simulink model "MCU_Input"  (R2022b)
settings: Solver=FixedStepDiscrete  StartTime=0.0  StopTime=10.0  FixedStep=1e-4  RelTol=1e-3
values from neighbouring files (symbols this model uses):
  C_ADC_Acc1Offset_i32 = 0.0    [MCU_Input_Sldd.sldd]    (also in MCU_Input_Sldd_objects.m = myPackage.Parameter)
  C_ADC_BrakeOffset_i32 = 0.0    [MCU_Input_Sldd.sldd]    (also in MCU_Input_Sldd_objects.m = myPackage.Parameter)
  C_ADC_HSTempGain_f32 = 0.0    [MCU_Input_Sldd.sldd]    (also in MCU_Input_Sldd_objects.m = myPackage.Parameter)
  C_ADC_HSTempOffset_i32 = 0.0    [MCU_Input_Sldd.sldd]    (also in MCU_Input_Sldd_objects.m = myPackage.Parameter)
  C_ADC_IdcOffset_i32 = 0.0    [MCU_Input_Sldd.sldd]    (also in MCU_Input_Sldd_objects.m = myPackage.Parameter)
  C_ADC_IGBTTable_i16 = 0.0    [MCU_Input_Sldd.sldd]    (also in MCU_Input_Sldd_objects.m = myPackage.Parameter)
  C_ADC_IGBTTempGain_f32 = 0.0    [MCU_Input_Sldd.sldd]    (also in MCU_Input_Sldd_objects.m = myPackage.Parameter)
  C_ADC_IGBTTempOffset_i32 = 0.0    [MCU_Input_Sldd.sldd]    (also in MCU_Input_Sldd_objects.m = myPackage.Parameter)
  C_ADC_MotorTemp1Gain_f32 = 0.0    [MCU_Input_Sldd.sldd]    (also in MCU_Input_Sldd_objects.m = myPackage.Parameter)
  C_ADC_MotorTemp1Offset_i32 = 0.0    [MCU_Input_Sldd.sldd]    (also in MCU_Input_Sldd_objects.m = myPackage.Parameter)
  C_ADC_MotorTempTable_i16 = 0.0    [MCU_Input_Sldd.sldd]    (also in MCU_Input_Sldd_objects.m = myPackage.Parameter)
  C_ADC_P12VOffset_i32 = 0.0    [MCU_Input_Sldd.sldd]    (also in MCU_Input_Sldd_objects.m = myPackage.Parameter)
  C_ADC_P15VOffset_i32 = 0.0    [MCU_Input_Sldd.sldd]    (also in MCU_Input_Sldd_objects.m = myPackage.Parameter)
  C_ADC_P5VOffset_i32 = 0.0    [MCU_Input_Sldd.sldd]    (also in MCU_Input_Sldd_objects.m = myPackage.Parameter)
  C_DCCurrent_DrvCoeff_f32 = 0.0    [MCU_Input_Sldd.sldd]    (also in MCU_Input_Sldd_objects.m = myPackage.Parameter)
  C_DCCurrent_GenCoeff_f32 = 0.0    [MCU_Input_Sldd.sldd]    (also in MCU_Input_Sldd_objects.m = myPackage.Parameter)
  C_Encoder_CurrentAdder_f32 = 0.0    [MCU_Input_Sldd.sldd]    (also in MCU_Input_Sldd_objects.m = myPackage.Parameter)
  C_Encoder_WaitTime_f32 = 0.0    [MCU_Input_Sldd.sldd]    (also in MCU_Input_Sldd_objects.m = myPackage.Parameter)
  C_Input_EncErr_u8 = 0.0    [MCU_Input_Sldd.sldd]    (also in MCU_Input_Sldd_objects.m = myPackage.Parameter)
  C_Rotate_RotateBits_u8 = 0.0    [MCU_Input_Sldd.sldd]    (also in MCU_Input_Sldd_objects.m = myPackage.Parameter)
  C_Rotate_SetAngle_u16 = 0.0    [MCU_Input_Sldd.sldd]    (also in MCU_Input_Sldd_objects.m = myPackage.Parameter)
  C_Rotate_SetAngleFlg_u8 = 0.0    [MCU_Input_Sldd.sldd]    (also in MCU_Input_Sldd_objects.m = myPackage.Parameter)
  C_SelfCheck_AvgCntSet_u16 = 0.0    [MCU_Input_Sldd.sldd]    (also in MCU_Input_Sldd_objects.m = myPackage.Parameter)
  C_SelfCheck_DelayTimeSet_u16 = 0.0    [MCU_Input_Sldd.sldd]    (also in MCU_Input_Sldd_objects.m = myPackage.Parameter)
  C_SelfCheck_IaoffsetDownLimt_u16 = 0.0    [MCU_Input_Sldd.sldd]    (also in MCU_Input_Sldd_objects.m = myPackage.Parameter)
  C_SelfCheck_IaoffsetUpLimt_u16 = 0.0    [MCU_Input_Sldd.sldd]    (also in MCU_Input_Sldd_objects.m = myPackage.Parameter)
  C_SelfCheck_IboffsetDownLimt_u16 = 0.0    [MCU_Input_Sldd.sldd]    (also in MCU_Input_Sldd_objects.m = myPackage.Parameter)
  C_SelfCheck_IboffsetUpLimt_u16 = 0.0    [MCU_Input_Sldd.sldd]    (also in MCU_Input_Sldd_objects.m = myPackage.Parameter)
  C_SelfCheck_IcoffsetDownLimt_u16 = 0.0    [MCU_Input_Sldd.sldd]    (also in MCU_Input_Sldd_objects.m = myPackage.Parameter)
  C_SelfCheck_IcoffsetUpLimt_u16 = 0.0    [MCU_Input_Sldd.sldd]    (also in MCU_Input_Sldd_objects.m = myPackage.Parameter)
  C_SelfCheck_OffsetUnCal_u8 = 0.0    [MCU_Input_Sldd.sldd]    (also in MCU_Input_Sldd_objects.m = myPackage.Parameter)
undefined symbols (not defined in the file or in its folder): AB_SAMPLE, ABC_SAMPLE, AC_SAMPLE, ANALOG, BC_SAMPLE, cAgeingMode, cParaRecogMode, cVvvfOpenMode, ParamCfg_AdAcc1K_u16, ParamCfg_AdBrakeK_u16, ParamCfg_AdIaK_u16, ParamCfg_AdIbK_u16, ParamCfg_AdIcK_u16, ParamCfg_AdKeyK_u16, ParamCfg_AdP12vK_u16, ParamCfg_AdP15vK_u16, ParamCfg_AdP5vK_u16, ParamCfg_AdUdcK_u16, ParamCfg_AdVonK_u16, ParamCfg_Avgcnt_u16, ParamCfg_BaseCur_u16, ParamCfg_BaseUdc_u16, ParamCfg_CommandSource_u16, ParamCfg_MaxSpeed_u16, ParamCfg_MotorNp_u16, ParamCfg_PosInit_u16, ParamCfg_PowerMax_u16, ParamCfg_PwmFreqLow_u16, ParamCfg_RotateDir_u16, ParamCfg_RotateNp_u16, ParamCfg_SampleMode_u16, ParamCfg_SensorSpeed_u16, ParamCfg_SmoPllKi_u16, ParamCfg_SmoPllKp_u16, ParamCfg_Stage_u16, ParamCfg_ThetaGain_u16, ParamCfg_UdcDefValue_u16, POWER_ON, STANDBY
libraries: simulink x41, YS_UserDefined_Library x4
(part 5 of 5)

== stateflow chart MCU_Input/Input_100us/Rotate_100us/RotateCalc/En/Chart/PosLimit/LimitChart ==
  (default) -> (junction 3)
  (junction 3) -> (junction 5) [order 1] : [Pos > MaxPos]
  (junction 3) -> (junction 12) [order 2]
  (junction 5) -> (junction 7) : {tmpPos = Pos-MaxPos}
  (junction 7) -> (junction 10)
  (junction 10) -> (junction 40)
  (junction 12) -> (junction 20) [order 1]
  (junction 20) -> (junction 14) [order 1] : [Pos < 0]
  (junction 12) -> (junction 31) [order 2]
  (junction 20) -> (junction 23) [order 2]
  (junction 14) -> (junction 16)
  (junction 16) -> (junction 18) : {tmpPos = Pos+MaxPos}
  (junction 18) -> (junction 29)
  (junction 23) -> (junction 27) [order 1] : {tmpPos = Pos}
  (junction 23) -> (junction 36) [order 2]
  (junction 27) -> (junction 33)
  (junction 36) -> (junction 31)
  (junction 33) -> (junction 36)
  (junction 29) -> (junction 33)
  (junction 31) -> (junction 42)
  (junction 40) -> (junction 42)
  (junction 42) -> (junction 45)
  data: Pos input int16; MaxPos input uint16; tmpPos output int16 =0
